simulink model "sim4_laboratorium"  (R2023b)
settings: Solver=VariableStepAuto  StartTime=0.0  StopTime=10.0  RelTol=1e-3
values from neighbouring files (symbols this model uses):
  c_denom = [ 1, 3, 3, 1]    [zadanie3.m]
  c_nom = [ 0, 0, 0, 1 ]    [zadanie3.m]
  final_value = 1    [zadanie3.m]
  init_value = 0    [zadanie3.m]
  pi_cont_denom = [ 1, 0]    [zadanie3.m]
  pi_cont_nom = [ kp, ki ]    [zadanie3.m]
  time_step = 0    [zadanie3.m]
settings Model: Creator=tomasz  LastModifiedBy=tomasz

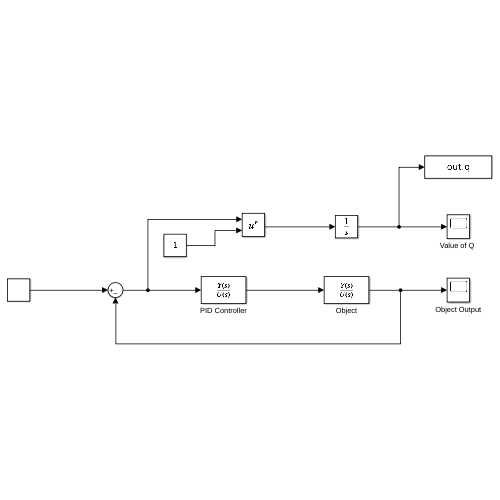
[thumbnail: Simulink's stored preview of the top-level diagram]
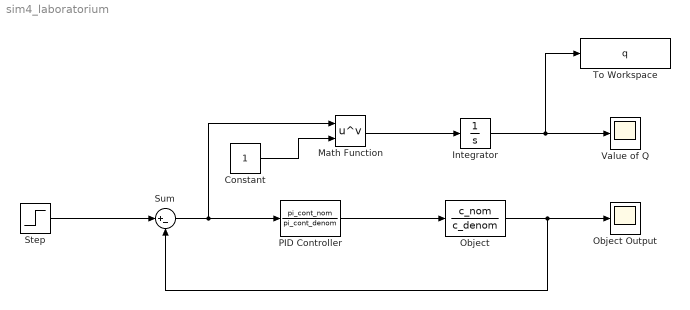
== system sim4_laboratorium ==
  Constant : Constant
  Integrator : Integrator
  Math Function : Math  Operator=pow
  Object : TransferFcn  Numerator=c_nom  Denominator=c_denom
  Object Output : Scope
  PID Controller : TransferFcn  Numerator=pi_cont_nom  Denominator=pi_cont_denom
  Step : Step  Time=time_step  Before=init_value  After=final_value  SampleTime=0
  Sum : Sum  Inputs=|+-
  To Workspace : ToWorkspace  VariableName=q  SaveFormat=Timeseries  SampleTime=-1
  "Value of Q " : Scope
  wires:
  Sum/1 -> Math Function/1, PID Controller/1
  PID Controller/1 -> Object/1
  Object/1 -> Sum/2, Object Output/1
  Step/1 -> Sum/1
  Constant/1 -> Math Function/2
  Math Function/1 -> Integrator/1
  Integrator/1 -> To Workspace/1, "Value of Q "/1
